simulink model "Running_mex_SIMULINK"  (R2020a)
settings: Solver=VariableStepAuto  StartTime=0.0  StopTime=inf  RelTol=1e-3
values from neighbouring files (symbols this model uses):
  angdes = fliplr(angdes)    [running_simulink_function_stepsize.m]    (also in simulink_run_file.m)
  C1 = inputs(end-6:end-4)    [linearize_get_Gain.m]    (also in running_simulink_function_stepsize.m = [70,15,15]; simulink_run_file.m = [1,1,1])
  C2 = inputs(end-3:end-1)    [linearize_get_Gain.m]    (also in running_simulink_function_stepsize.m = [.01,7,15]; simulink_run_file.m = [150,110,150])
  R = inputs(end)    [linearize_get_Gain.m]    (also in running_simulink_function_stepsize.m = 500; simulink_run_file.m = 1000000)
  refresh = .001    (= 0.001)    [simulink_run_file.m]
  Tfinal_master = refresh*NumSteps    [running_simulink_function_stepsize.m]    (also in simulink_run_file.m)
  Tmax = 2/1000    (= 0.002)    [running_simulink_function_stepsize.m]    (also in simulink_run_file.m)
  U4des = 0    [running_simulink_function_stepsize.m]    (also in simulink_run_file.m)
  U5des = 0    [running_simulink_function_stepsize.m]    (also in simulink_run_file.m)
  U6des = 0    [running_simulink_function_stepsize.m]    (also in simulink_run_file.m)
undefined symbols (not defined in the file or in its folder): get_initial_inputs
settings Model: Creator=hoddid  LastModifiedBy=hoddid

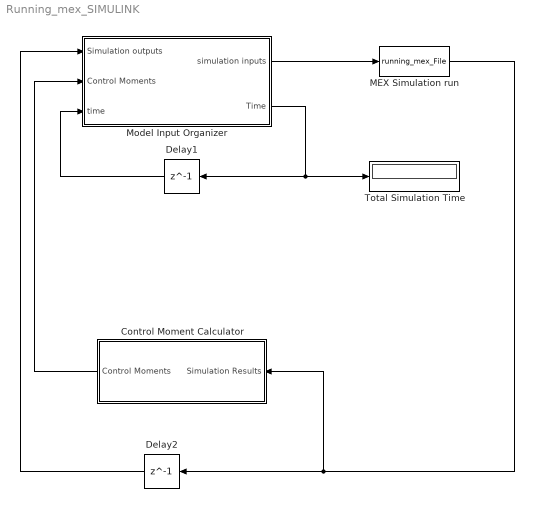
== system Running_mex_SIMULINK ==
  Control Moment Calculator : Subsystem
  Delay1 : Delay  DelayLength=1
  Delay2 : Delay  DelayLength=1
  MEX Simulation run : MATLABFcn  MATLABFcn=running_mex_File  OutputDimensions=[1 32]  Output1D=off
  Model Input Organizer : Subsystem
  Total Simulation Time : Display
  wires:
  Model Input Organizer/1(simulation inputs) -> MEX Simulation run/1
  MEX Simulation run/1 -> Delay2/1, Control Moment Calculator/1(Simulation Results)
  Delay1/1 -> Model Input Organizer/3(time)
  Control Moment Calculator/1(Control Moments) -> Model Input Organizer/2(Control Moments)
  Model Input Organizer/2(Time) -> Delay1/1, Total Simulation Time/1
  Delay2/1 -> Model Input Organizer/1(Simulation outputs)

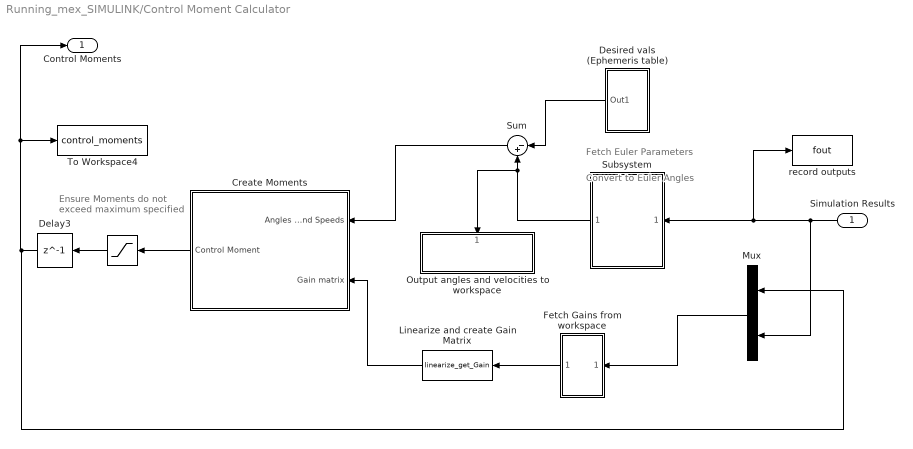
== system Running_mex_SIMULINK/Control Moment Calculator ==
  note: Ensure Moments do not
      | exceed maximum specified
  note: Fetch Euler Parameters
  note: Convert to Euler Angles
  Simulation Results : Inport
  " " : Saturate  UpperLimit=Tmax  LowerLimit=-Tmax
  Create Moments : Subsystem
  Delay3 : Delay  DelayLength=1
  Desired vals (Ephemeris table) : Subsystem
  Fetch Gains from workspace : Subsystem
  Linearize and create Gain Matrix : MATLABFcn  MATLABFcn=linearize_get_Gain  OutputDimensions=[3 6]  Output1D=off
  Mux : Mux  Inputs=2
  Output angles and velocities to workspace : Subsystem
      settings: PortSchema="{\"entries\":[{\"content\":{\"sides\":[{\"content\":{\"connectorIds\":[]},\"type\":\"ConnectorPlacement.EquallySpacedRectSide\",\"uuid\":\"710fda5a-db72-41f7-ab86-ad5d4ff48fe3\"},{\"content\":{\"connectorIds\":[],\"side\":\"RIGHT\"},\"type\":\"ConnectorPlacement.EquallySpacedRectSide\",\"uuid\":\"920054e7-8472-4e0a-919a-5b3769e7d821\"},{\"content\":{\"connectorIds\":[\"In1\"],\"side\":\"TOP\"},\"type\":\"ConnectorPlacement.EquallySpacedRectSide\",\"uuid\":\"b1b8d1a9-336f-4444-a2e2-06c501d100f8\"}]},\"type\":\"ConnectorPlacement.EquallySpacedConnector\",\"uuid\":\"8db0526a-99ef-4736-81ba-f5f4ce7ad37f\"}],\"packageUris\":[\"http://schema.mathworks.com/mf0/Connector/19700101\"],\"version\":\"1.0\"}"
  Subsystem : Subsystem
  Sum : Sum  Inputs=|-+
  To Workspace4 : ToWorkspace  VariableName=control_moments  SampleTime=-1
      settings: Save2DSignal=2-D array (concatenate along first dimension)
  record outputs : ToWorkspace  VariableName=fout  SampleTime=-1
      settings: Save2DSignal=2-D array (concatenate along first dimension)
  Control Moments : Outport
  wires:
  Mux/1 -> Fetch Gains from workspace/1(In1)
  Linearize and create Gain Matrix/1 -> Create Moments/2(Gain matrix)
  Simulation Results/1 -> Mux/2, record outputs/1, Subsystem/1(last_results)
  Fetch Gains from workspace/1(Out1) -> Linearize and create Gain Matrix/1
  Delay3/1 -> Control Moments/1, To Workspace4/1, Mux/1
  Subsystem/1(Output) -> Output angles and velocities to workspace/1(1), Sum/2
  Desired vals (Ephemeris table)/1(Out1) -> Sum/1
  Sum/1 -> Create Moments/1(Angles and Speeds)
  " "/1 -> Delay3/1
  Create Moments/1(Control Moment) -> " "/1

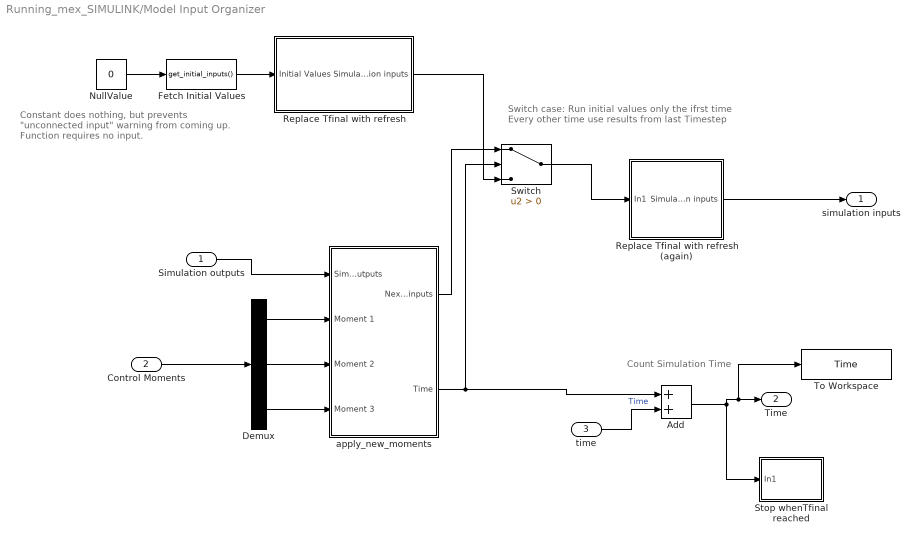
== system Running_mex_SIMULINK/Model Input Organizer ==
  note: Count Simulation Time
  note: Switch case: Run initial values only the ifrst time
      | Every other time use results from last Timestep
  note: Constant does nothing, but prevents
      | "unconnected input" warning from coming up.
      | Function requires no input.
  Simulation outputs : Inport
  Control Moments : Inport  Port=2
  time : Inport  Port=3
  Add : Sum
  Demux : Demux  Outputs=3
  Fetch Initial Values : MATLABFcn  MATLABFcn=get_initial_inputs()
  NullValue : Constant  Value=0
  Replace Tfinal with refresh : Subsystem
  Replace Tfinal with refresh (again) : Subsystem
  Stop whenTfinal reached : Subsystem
      settings: PortSchema="{\"entries\":[{\"content\":{\"sides\":[{\"content\":{\"connectorIds\":[]},\"type\":\"ConnectorPlacement.EquallySpacedRectSide\",\"uuid\":\"b8031d13-d17c-4f9a-b5f8-92da6927a3ba\"},{\"content\":{\"connectorIds\":[],\"side\":\"RIGHT\"},\"type\":\"ConnectorPlacement.EquallySpacedRectSide\",\"uuid\":\"11a71682-1cdb-45f2-b8b8-d175538f4c28\"},{\"content\":{\"connectorIds\":[\"In1\"],\"side\":\"TOP\"},\"type\":\"ConnectorPlacement.EquallySpacedRectSide\",\"uuid\":\"ae57efda-2ecd-443a-aa6f-cfe1c35dec26\"}]},\"type\":\"ConnectorPlacement.EquallySpacedConnector\",\"uuid\":\"64a769af-a08f-48b5-9fd8-ee733c537d04\"}],\"packageUris\":[\"http://schema.mathworks.com/mf0/Connector/19700101\"],\"version\":\"1.0\"}"
  Switch : Switch  Criteria=u2 > Threshold
  To Workspace : ToWorkspace  VariableName=Time  SampleTime=-1
      settings: Save2DSignal=2-D array (concatenate along first dimension)
  apply_new_moments : Subsystem
  simulation inputs : Outport
  Time : Outport  Port=2
  wires:
  Simulation outputs/1 -> apply_new_moments/1(Simulation outputs)
  apply_new_moments/1(Next Simulation inputs) -> Switch/1
  apply_new_moments/2(Time) -> Add/1, Switch/2
  time/1 -> Add/2  "Time"
  Add/1 -> To Workspace/1, Time/1, Stop whenTfinal reached/1(In1)
  Switch/1 -> Replace Tfinal with refresh (again)/1(In1)
  Fetch Initial Values/1 -> Replace Tfinal with refresh/1(Initial Values)
  Replace Tfinal with refresh/1(Simulation inputs) -> Switch/3
  Replace Tfinal with refresh (again)/1(Simulation inputs) -> simulation inputs/1
  NullValue/1 -> Fetch Initial Values/1
  Control Moments/1 -> Demux/1
  Demux/1 -> apply_new_moments/2(Moment 1)
  Demux/2 -> apply_new_moments/3(Moment 2)
  Demux/3 -> apply_new_moments/4(Moment 3)

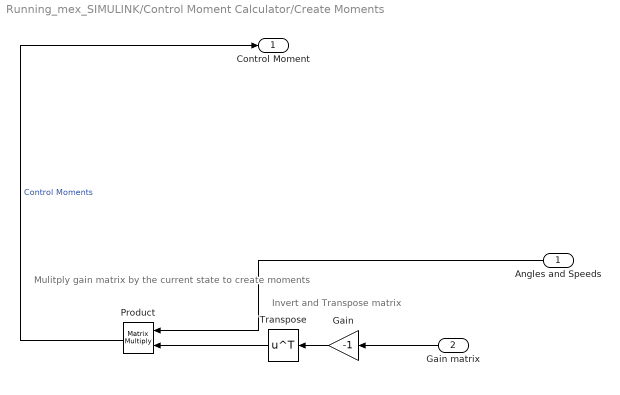
== system Running_mex_SIMULINK/Control Moment Calculator/Create Moments ==
  note: Mulitply gain matrix by the current state to create moments
  note: Invert and Transpose matrix
  Angles and Speeds : Inport
  Gain matrix : Inport  Port=2
  Gain : Gain  Gain=-1
  Product : Product  Multiplication=Matrix(*)
  Transpose : Math  Operator=transpose  SaturateOnIntegerOverflow=on
  Control Moment : Outport
  wires:
  Gain/1 -> Transpose/1
  Product/1 -> Control Moment/1  "Control Moments"
  Gain matrix/1 -> Gain/1
  Angles and Speeds/1 -> Product/1
  Transpose/1 -> Product/2

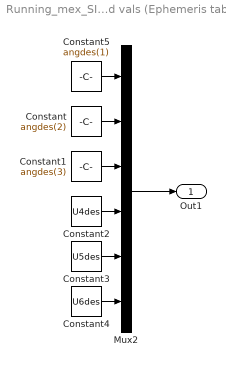
== system Running_mex_SIMULINK/Control Moment Calculator/Desired vals (Ephemeris table) ==
  Constant : Constant  Value=angdes(2)
  Constant1 : Constant  Value=angdes(3)
  Constant2 : Constant  Value=U4des
  Constant3 : Constant  Value=U5des
  Constant4 : Constant  Value=U6des
  Constant5 : Constant  Value=angdes(1)
  Mux2 : Mux  Inputs=6
  Out1 : Outport
  wires:
  Constant1/1 -> Mux2/3
  Constant3/1 -> Mux2/5
  Constant5/1 -> Mux2/1
  Mux2/1 -> Out1/1
  Constant/1 -> Mux2/2
  Constant4/1 -> Mux2/6
  Constant2/1 -> Mux2/4

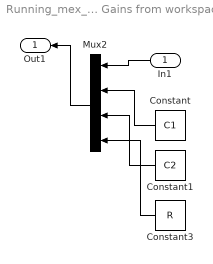
== system Running_mex_SIMULINK/Control Moment Calculator/Fetch Gains from workspace ==
  In1 : Inport
  Constant : Constant  Value=C1
  Constant1 : Constant  Value=C2
  Constant3 : Constant  Value=R
  Mux2 : Mux
  Out1 : Outport
  wires:
  Constant3/1 -> Mux2/4
  Constant1/1 -> Mux2/3
  Mux2/1 -> Out1/1
  In1/1 -> Mux2/1
  Constant/1 -> Mux2/2

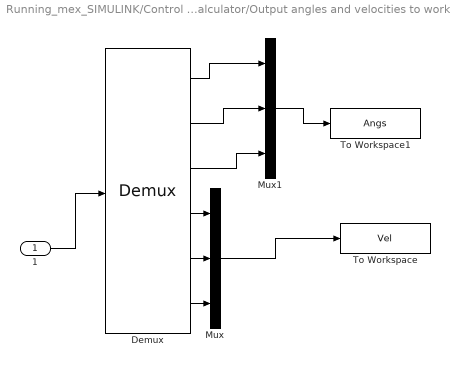
== system Running_mex_SIMULINK/Control Moment Calculator/Output angles and velocities to workspace ==
  1 : Inport
  Demux : Demux  Outputs=6
  Mux : Mux  Inputs=3
  Mux1 : Mux  Inputs=3
  To Workspace : ToWorkspace  VariableName=Vel  SampleTime=-1
      settings: Save2DSignal=2-D array (concatenate along first dimension)
  To Workspace1 : ToWorkspace  VariableName=Angs  SampleTime=-1
      settings: Save2DSignal=2-D array (concatenate along first dimension)
  wires:
  1/1 -> Demux/1
  Demux/4 -> Mux/1
  Demux/5 -> Mux/2
  Demux/6 -> Mux/3
  Mux/1 -> To Workspace/1
  Demux/1 -> Mux1/1
  Demux/2 -> Mux1/2
  Demux/3 -> Mux1/3
  Mux1/1 -> To Workspace1/1

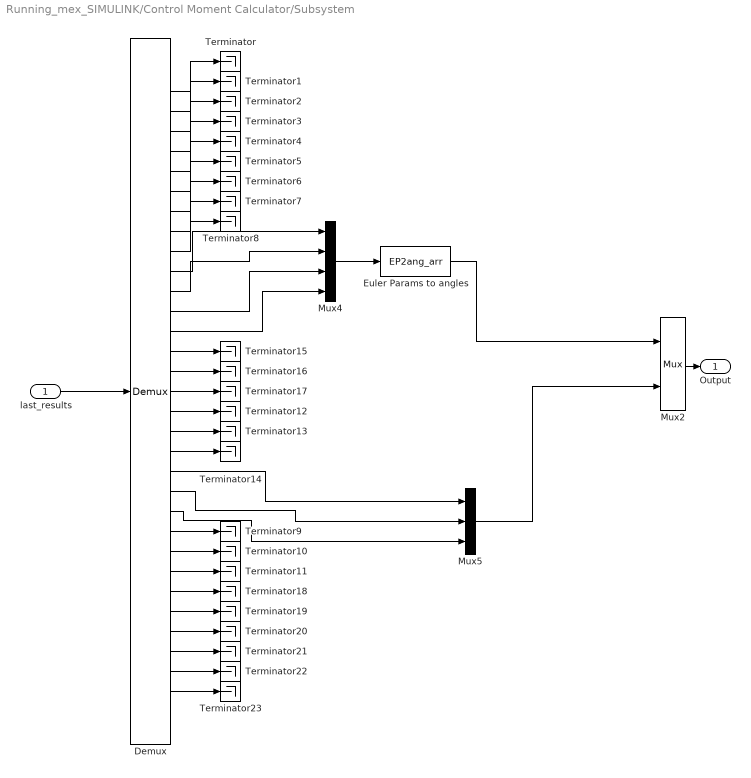
== system Running_mex_SIMULINK/Control Moment Calculator/Subsystem ==
  last_results : Inport
  Demux : Demux  Outputs=31
  Euler Params to angles : MATLABFcn  MATLABFcn=EP2ang_arr
  Mux2 : Mux  Inputs=2
  Mux4 : Mux
  Mux5 : Mux  Inputs=3
  Terminator{,1..23} (24 alike) : Terminator
  Output : Outport  PortDimensions=[1 6]
  wires:
  last_results/1 -> Demux/1
  Mux4/1 -> Euler Params to angles/1
  Mux5/1 -> Mux2/2
  Mux2/1 -> Output/1
  Demux/1 -> Terminator/1
  Demux/2 -> Terminator1/1
  Demux/3 -> Terminator2/1
  Demux/4 -> Terminator3/1
  Demux/5 -> Terminator4/1
  Demux/6 -> Terminator5/1
  Demux/9 -> Terminator8/1
  Demux/7 -> Terminator6/1
  Demux/8 -> Terminator7/1
  Demux/12 -> Mux4/3
  Demux/10 -> Mux4/1
  Demux/11 -> Mux4/2
  Demux/19 -> Terminator14/1
  Demux/17 -> Terminator12/1
  Demux/18 -> Terminator13/1
  Demux/22 -> Mux5/3
  Demux/20 -> Mux5/1
  Demux/21 -> Mux5/2
  Demux/28 -> Terminator20/1
  Demux/26 -> Terminator18/1
  Demux/27 -> Terminator19/1
  Demux/31 -> Terminator23/1
  Demux/29 -> Terminator21/1
  Demux/30 -> Terminator22/1
  Demux/13 -> Mux4/4
  Demux/24 -> Terminator10/1
  Demux/23 -> Terminator9/1
  Demux/25 -> Terminator11/1
  Demux/15 -> Terminator16/1
  Demux/14 -> Terminator15/1
  Demux/16 -> Terminator17/1
  Euler Params to angles/1 -> Mux2/1

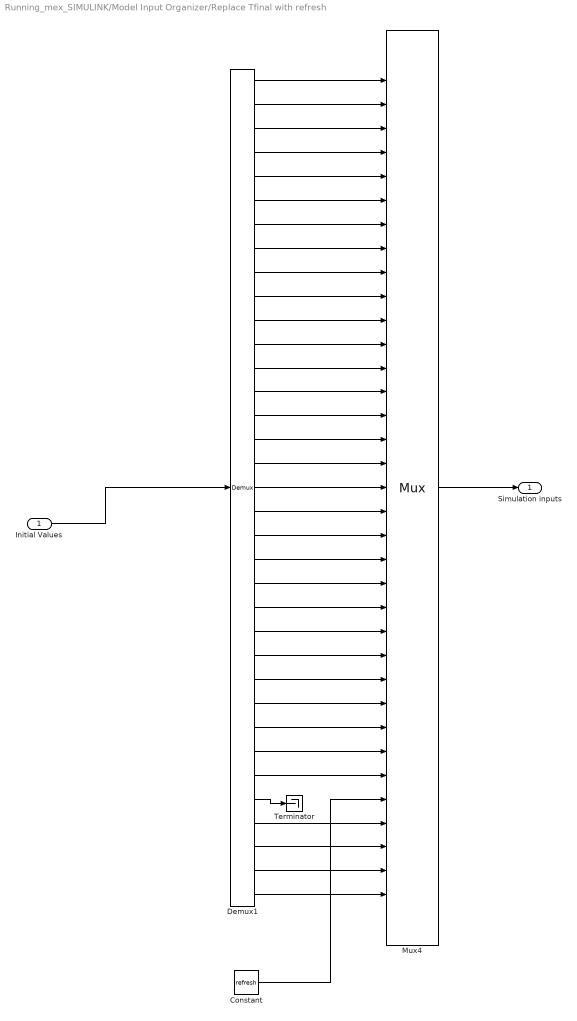
== system Running_mex_SIMULINK/Model Input Organizer/Replace Tfinal with refresh ==
  Initial Values : Inport
  Constant : Constant  Value=refresh
  Demux1 : Demux  Outputs=35
  Mux4 : Mux  Inputs=35
  Terminator : Terminator
  Simulation inputs : Outport  OutDataTypeStr=double
  wires:
  Initial Values/1 -> Demux1/1
  Mux4/1 -> Simulation inputs/1
  Demux1/1 -> Mux4/1
  Demux1/2 -> Mux4/2
  Demux1/3 -> Mux4/3
  Demux1/4 -> Mux4/4
  Demux1/5 -> Mux4/5
  Demux1/6 -> Mux4/6
  Demux1/7 -> Mux4/7
  Demux1/8 -> Mux4/8
  Demux1/9 -> Mux4/9
  Demux1/10 -> Mux4/10
  Demux1/11 -> Mux4/11
  Demux1/12 -> Mux4/12
  Demux1/13 -> Mux4/13
  Demux1/14 -> Mux4/14
  Demux1/15 -> Mux4/15
  Demux1/16 -> Mux4/16
  Demux1/17 -> Mux4/17
  Demux1/18 -> Mux4/18
  Demux1/19 -> Mux4/19
  Demux1/20 -> Mux4/20
  Demux1/21 -> Mux4/21
  Demux1/22 -> Mux4/22
  Demux1/23 -> Mux4/23
  Demux1/24 -> Mux4/24
  Demux1/25 -> Mux4/25
  Demux1/26 -> Mux4/26
  Demux1/27 -> Mux4/27
  Demux1/28 -> Mux4/28
  Demux1/29 -> Mux4/29
  Constant/1 -> Mux4/31
  Demux1/31 -> Terminator/1
  Demux1/35 -> Mux4/35
  Demux1/34 -> Mux4/34
  Demux1/33 -> Mux4/33
  Demux1/32 -> Mux4/32
  Demux1/30 -> Mux4/30

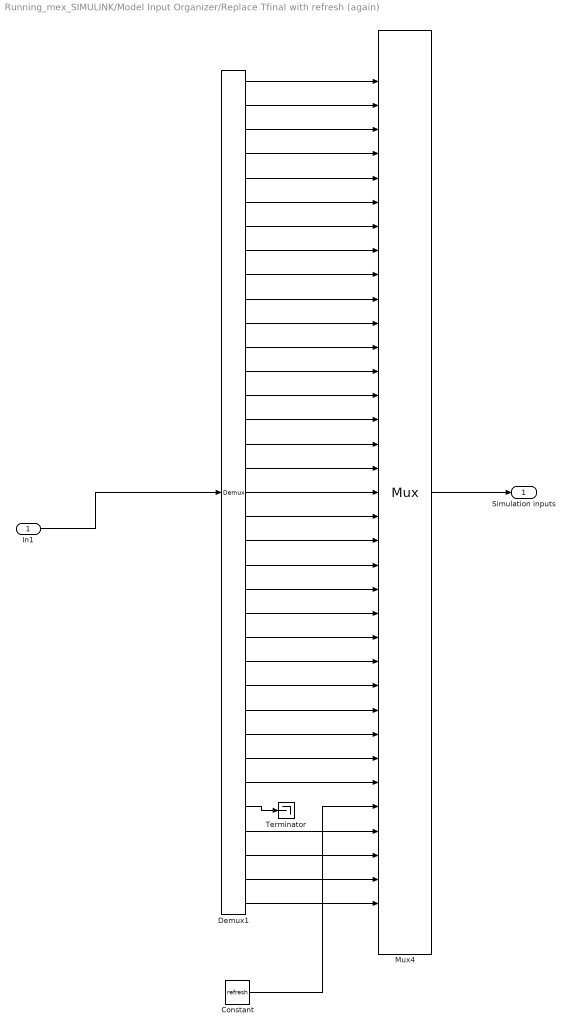
== system Running_mex_SIMULINK/Model Input Organizer/Replace Tfinal with refresh (again) ==
  In1 : Inport
  Constant : Constant  Value=refresh
  Demux1 : Demux  Outputs=35
  Mux4 : Mux  Inputs=35
  Terminator : Terminator
  Simulation inputs : Outport  OutDataTypeStr=double
  wires:
  In1/1 -> Demux1/1
  Mux4/1 -> Simulation inputs/1
  Demux1/1 -> Mux4/1
  Demux1/2 -> Mux4/2
  Demux1/3 -> Mux4/3
  Demux1/4 -> Mux4/4
  Demux1/5 -> Mux4/5
  Demux1/6 -> Mux4/6
  Demux1/7 -> Mux4/7
  Demux1/8 -> Mux4/8
  Demux1/9 -> Mux4/9
  Demux1/10 -> Mux4/10
  Demux1/11 -> Mux4/11
  Demux1/12 -> Mux4/12
  Demux1/13 -> Mux4/13
  Demux1/14 -> Mux4/14
  Demux1/15 -> Mux4/15
  Demux1/16 -> Mux4/16
  Demux1/17 -> Mux4/17
  Demux1/18 -> Mux4/18
  Demux1/19 -> Mux4/19
  Demux1/20 -> Mux4/20
  Demux1/21 -> Mux4/21
  Demux1/22 -> Mux4/22
  Demux1/23 -> Mux4/23
  Demux1/24 -> Mux4/24
  Demux1/25 -> Mux4/25
  Demux1/26 -> Mux4/26
  Demux1/27 -> Mux4/27
  Demux1/28 -> Mux4/28
  Demux1/29 -> Mux4/29
  Constant/1 -> Mux4/31
  Demux1/31 -> Terminator/1
  Demux1/35 -> Mux4/35
  Demux1/34 -> Mux4/34
  Demux1/33 -> Mux4/33
  Demux1/32 -> Mux4/32
  Demux1/30 -> Mux4/30

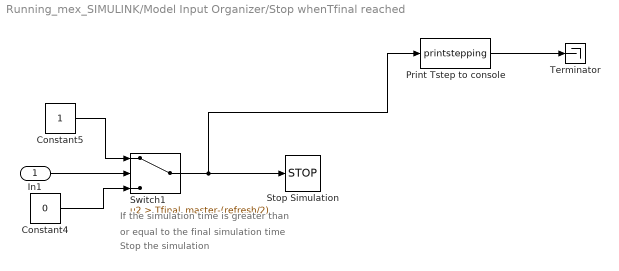
== system Running_mex_SIMULINK/Model Input Organizer/Stop whenTfinal reached ==
  note: Stop the simulation
  note: or equal to the final simulation time
  note: If the simulation time is greater than
  In1 : Inport
  Constant4 : Constant  Value=0
  Constant5 : Constant
  Print Tstep to console : MATLABFcn  MATLABFcn=printstepping
  Stop Simulation : Stop
  Switch1 : Switch  Criteria=u2 > Threshold  Threshold=Tfinal_master-(refresh/2)
  Terminator : Terminator
  wires:
  Constant4/1 -> Switch1/3
  In1/1 -> Switch1/2
  Switch1/1 -> Print Tstep to console/1, Stop Simulation/1
  Constant5/1 -> Switch1/1
  Print Tstep to console/1 -> Terminator/1

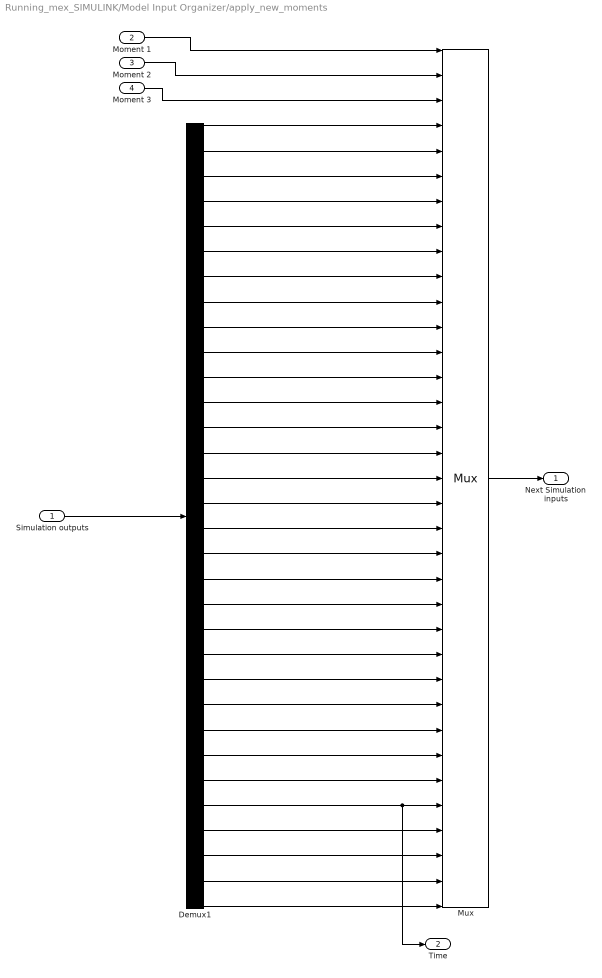
== system Running_mex_SIMULINK/Model Input Organizer/apply_new_moments ==
  Simulation outputs : Inport
  Moment 1 : Inport  Port=2
  Moment 2 : Inport  Port=3
  Moment 3 : Inport  Port=4
  Demux1 : Demux  Outputs=32
  Mux : Mux  Inputs=35
  Next Simulation inputs : Outport  OutDataTypeStr=double
  Time : Outport  Port=2
  wires:
  Simulation outputs/1 -> Demux1/1
  Moment 3/1 -> Mux/3
  Moment 2/1 -> Mux/2
  Moment 1/1 -> Mux/1
  Mux/1 -> Next Simulation inputs/1
  Demux1/1 -> Mux/4
  Demux1/2 -> Mux/5
  Demux1/3 -> Mux/6
  Demux1/4 -> Mux/7
  Demux1/5 -> Mux/8
  Demux1/6 -> Mux/9
  Demux1/7 -> Mux/10
  Demux1/8 -> Mux/11
  Demux1/9 -> Mux/12
  Demux1/10 -> Mux/13
  Demux1/11 -> Mux/14
  Demux1/12 -> Mux/15
  Demux1/13 -> Mux/16
  Demux1/14 -> Mux/17
  Demux1/15 -> Mux/18
  Demux1/16 -> Mux/19
  Demux1/17 -> Mux/20
  Demux1/18 -> Mux/21
  Demux1/19 -> Mux/22
  Demux1/20 -> Mux/23
  Demux1/21 -> Mux/24
  Demux1/22 -> Mux/25
  Demux1/23 -> Mux/26
  Demux1/24 -> Mux/27
  Demux1/25 -> Mux/28
  Demux1/26 -> Mux/29
  Demux1/27 -> Mux/30
  Demux1/28 -> Time/1, Mux/31
  Demux1/29 -> Mux/32
  Demux1/30 -> Mux/33
  Demux1/31 -> Mux/34
  Demux1/32 -> Mux/35
